simulink model "Comprobacion"  (R2024b)
settings: Solver=VariableStepAuto  StartTime=0.0  StopTime=10.0  RelTol=1e-3
settings Model: Creator=javier  LastModifiedBy=javier

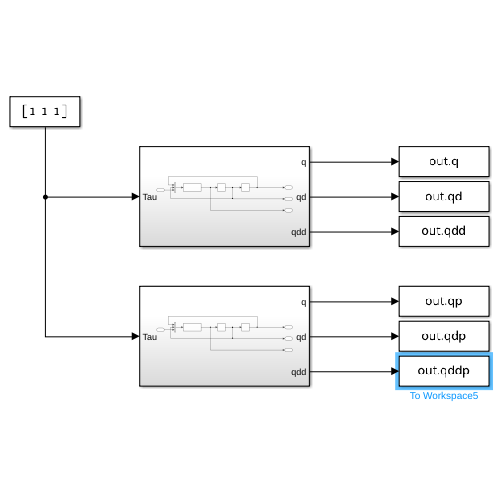
[thumbnail: Simulink's stored preview of the top-level diagram]
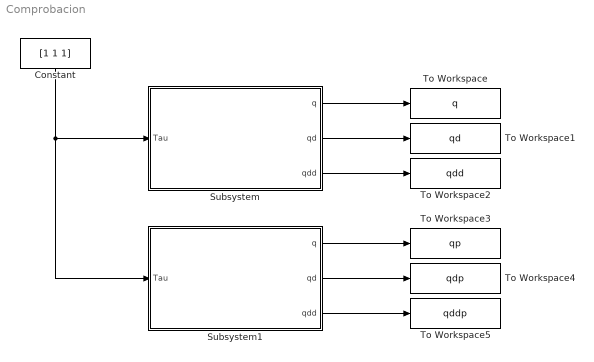
== system Comprobacion ==
  Constant : Constant  Value=[1 1 1]
  Subsystem : Subsystem
  Subsystem1 : Subsystem
  To Workspace : ToWorkspace  VariableName=q  SampleTime=-1
  To Workspace1 : ToWorkspace  VariableName=qd  SampleTime=-1
  To Workspace2 : ToWorkspace  VariableName=qdd  SampleTime=-1
  To Workspace3 : ToWorkspace  VariableName=qp  SampleTime=-1
  To Workspace4 : ToWorkspace  VariableName=qdp  SampleTime=-1
  To Workspace5 : ToWorkspace  VariableName=qddp  SampleTime=-1
  wires:
  Constant/1 -> Subsystem1/1(Tau), Subsystem/1(Tau)
  Subsystem/1(q) -> To Workspace/1
  Subsystem/2(qd) -> To Workspace1/1
  Subsystem/3(qdd) -> To Workspace2/1
  Subsystem1/3(qdd) -> To Workspace5/1
  Subsystem1/1(q) -> To Workspace3/1
  Subsystem1/2(qd) -> To Workspace4/1

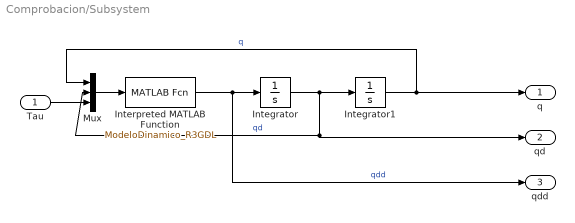
== system Comprobacion/Subsystem ==
  Tau : Inport
  Integrator : Integrator
  Integrator1 : Integrator
  Interpreted MATLAB Function : MATLABFcn  MATLABFcn=ModeloDinamico_R3GDL  OutputDimensions=3
  Mux : Mux  Inputs=3
  q : Outport
  qd : Outport  Port=2
  qdd : Outport  Port=3
  wires:
  Mux/1 -> Interpreted MATLAB Function/1
  Integrator/1 -> Mux/2, qd/1, Integrator1/1  "qd"
  Interpreted MATLAB Function/1 -> qdd/1, Integrator/1  "qdd"
  Integrator1/1 -> q/1, Mux/1  "q"
  Tau/1 -> Mux/3

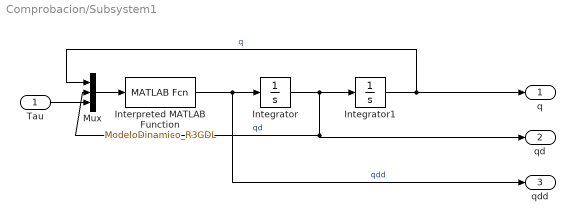
== system Comprobacion/Subsystem1 ==
  Tau : Inport
  Integrator : Integrator
  Integrator1 : Integrator
  Interpreted MATLAB Function : MATLABFcn  MATLABFcn=ModeloDinamico_R3GDL  OutputDimensions=3
  Mux : Mux  Inputs=3
  q : Outport
  qd : Outport  Port=2
  qdd : Outport  Port=3
  wires:
  Mux/1 -> Interpreted MATLAB Function/1
  Integrator/1 -> Mux/2, qd/1, Integrator1/1  "qd"
  Interpreted MATLAB Function/1 -> qdd/1, Integrator/1  "qdd"
  Integrator1/1 -> q/1, Mux/1  "q"
  Tau/1 -> Mux/3
